simulink model "Simulink10"  (Simulink 5.0)
settings: Solver=ode45  StartTime=0.0  StopTime=50.0  RelTol=1e-6  AbsTol=1e-6
libraries: simulink x1
settings Model: LastModifiedBy=stevel

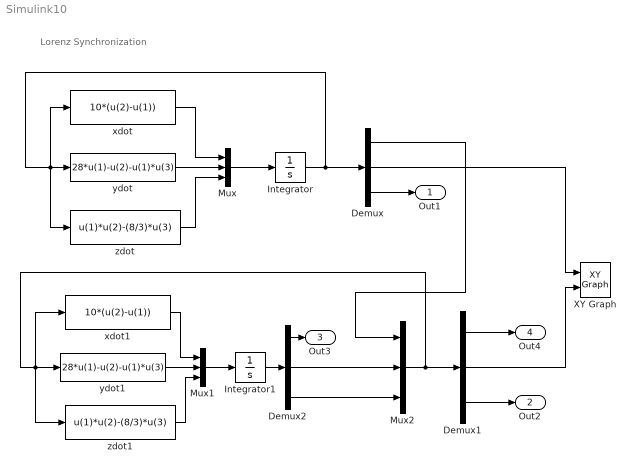
== system Simulink10 ==
  note: Lorenz Synchronization
  Demux : Demux  Outputs=3
  Demux1 : Demux  Outputs=3
  Demux2 : Demux  Outputs=3
  Integrator : Integrator  InitialCondition=[15 20 30]  UpperSaturationLimit=50  LowerSaturationLimit=0
  Integrator1 : Integrator  InitialCondition=[17 23 33]  UpperSaturationLimit=50  LowerSaturationLimit=0
  Mux : Mux  Inputs=3
  Mux1 : Mux  Inputs=3
  Mux2 : Mux  Inputs=3
  XY Graph : simulink/Sinks/XY Graph  xmin=-50  xmax=50  ymin=-50  ymax=50  st=-1
  xdot : Fcn  Description=sdhdkbkdf  Expr=10*(u(2)-u(1))
  xdot1 : Fcn  Description=sdhdkbkdf  Expr=10*(u(2)-u(1))
  ydot : Fcn  Expr=28*u(1)-u(2)-u(1)*u(3)
  ydot1 : Fcn  Expr=28*u(1)-u(2)-u(1)*u(3)
  zdot : Fcn  Expr=u(1)*u(2)-(8/3)*u(3)
  zdot1 : Fcn  Expr=u(1)*u(2)-(8/3)*u(3)
  Out1 : Outport
  Out2 : Outport  Port=2
  Out3 : Outport  Port=3
  Out4 : Outport  Port=4
  wires:
  xdot/1 -> Mux/1
  ydot/1 -> Mux/2
  zdot/1 -> Mux/3
  Mux/1 -> Integrator/1
  Integrator/1 -> ydot/1, xdot/1, zdot/1, Demux/1
  Demux/3 -> Out1/1
  xdot1/1 -> Mux1/1
  ydot1/1 -> Mux1/2
  zdot1/1 -> Mux1/3
  Mux2/1 -> Demux1/1, ydot1/1, xdot1/1, zdot1/1
  Demux1/3 -> Out2/1
  Demux/1 -> Mux2/1
  Mux1/1 -> Integrator1/1
  Integrator1/1 -> Demux2/1
  Demux2/2 -> Mux2/2
  Demux2/3 -> Mux2/3
  Demux2/1 -> Out3/1
  Demux/2 -> XY Graph/1
  Demux1/1 -> Out4/1
  Demux1/2 -> XY Graph/2
